simulink model "cascade_realization"  (R2020a)
settings: Solver=VariableStepAuto  StartTime=0.0  StopTime=10.0  RelTol=1e-3
settings Model: Creator=INDRAJIT MARATHE  LastModifiedBy=INDRAJIT MARATHE

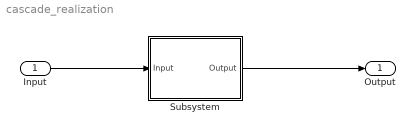
== system cascade_realization ==
  Input : Inport
  Subsystem : Subsystem  TreatAsAtomicUnit=on
  Output : Outport
  wires:
  Input/1 -> Subsystem/1(Input)
  Subsystem/1(Output) -> Output/1

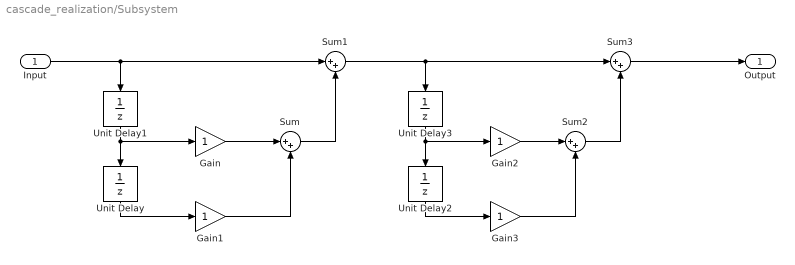
== system cascade_realization/Subsystem ==
  Input : Inport
  Gain{,1..3} (4 alike) : Gain
  Sum{,1..3} (4 alike) : Sum  Inputs=|++
  Unit Delay{,1..3} (4 alike) : UnitDelay  SampleTime=-1  HasFrameUpgradeWarning=on
  Output : Outport
  wires:
  Unit Delay1/1 -> Gain/1, Unit Delay/1
  Sum3/1 -> Output/1
  Sum1/1 -> Sum3/1, Unit Delay3/1
  Input/1 -> Sum1/1, Unit Delay1/1
  Gain1/1 -> Sum/2
  Unit Delay/1 -> Gain1/1
  Gain3/1 -> Sum2/2
  Sum/1 -> Sum1/2
  Gain/1 -> Sum/1
  Sum2/1 -> Sum3/2
  Unit Delay3/1 -> Gain2/1, Unit Delay2/1
  Gain2/1 -> Sum2/1
  Unit Delay2/1 -> Gain3/1
